simulink model "msync_foc"  (R2026a)
settings: Solver=ode15s  StopTime=t_sim  MaxStep=1e-4  MinStep=1e-8  RelTol=1e-4  AbsTol=1e-6
values from neighbouring files (symbols this model uses):
  f_frot = 1e-3    (= 0.001)    [init_machine_synchrone.m]
  Gamma_c = 1.0    (= 1)    [init_machine_synchrone.m]
  id_ref = 0    [init_machine_synchrone.m]
  Ir_ref = 4    [init_machine_synchrone.m]
  J = m*R^2/2    (= 0.246615023307)    [init_machine_synchrone.m]
  Ki_dq = Rs / tau_c    (= 1125)    [init_machine_synchrone.m]
  Ki_w = Kp_w / tau_w    (= 33891.230015)    [init_machine_synchrone.m]
  Kp_dq = Ls / tau_c    (= 15)    [init_machine_synchrone.m]
  Kp_w = J / (tau_w * M0 * Ir_ref)    (= 451.883066866)    [init_machine_synchrone.m]
  kr = ws_nom / t_rampe    (= 3.14159265359)    [init_machine_synchrone.m]
  Ls = 20e-3    (= 0.02)    [init_machine_synchrone.m]
  M0 = (V_ent/(2*mu0))*Ks*Kr    (= 0.010232805843)    [init_machine_synchrone.m]
  param_elec = [Rs ; Ls ; Rr ; Lr ; M0]    [init_machine_synchrone.m]
  Rr = 2.0    (= 2)    [init_machine_synchrone.m]
  theta0 = -pi/4    (= -0.785398163397)    [init_machine_synchrone.m]
  w0 = 0    [init_machine_synchrone.m]
  ws_nom = 2*pi*5    (= 31.4159265359)    [init_machine_synchrone.m]
  x_elec_0 = [i1_0; i2_0; Ir_0]    [init_machine_synchrone.m]
libraries: slpidlib x3, simulink x1
settings DebuggingCC: UnderSpecifiedDimensionMsg=warning

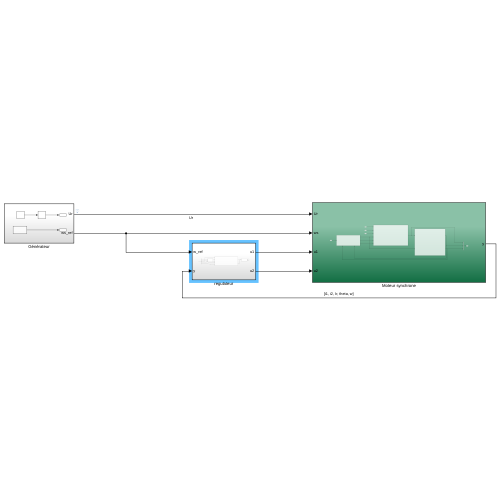
[thumbnail: Simulink's stored preview of the top-level diagram]
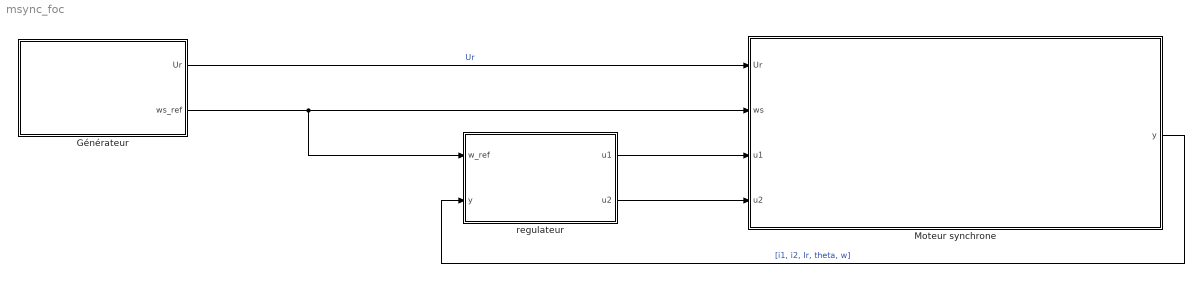
== system msync_foc ==
  Générateur : Subsystem
  Moteur synchrone : Subsystem
  regulateur : Subsystem
  wires:
  Générateur/1(Ur) -> Moteur synchrone/1(Ur)  "Ur"
  Générateur/2(ws_ref) -> Moteur synchrone/2(ws), regulateur/1(w_ref)
  regulateur/1(u1) -> Moteur synchrone/3(u1)
  regulateur/2(u2) -> Moteur synchrone/4(u2)
  Moteur synchrone/1(y) -> regulateur/2(y)  "[i1, i2, Ir, theta, w]"

== system msync_foc/Générateur ==
  Consigne rampe : simulink/Sources/Ramp  slope=kr  start=0  InitialOutput=20
  Constant : Constant  Value=Ir_ref/Rr
  Saturation : Saturate  UpperLimit=ws_nom  LowerLimit=-inf
  Ur : Outport
  ws_ref : Outport  Port=2
  wires:
  Constant/1 -> Ur/1
  Consigne rampe/1 -> Saturation/1
  Saturation/1 -> ws_ref/1

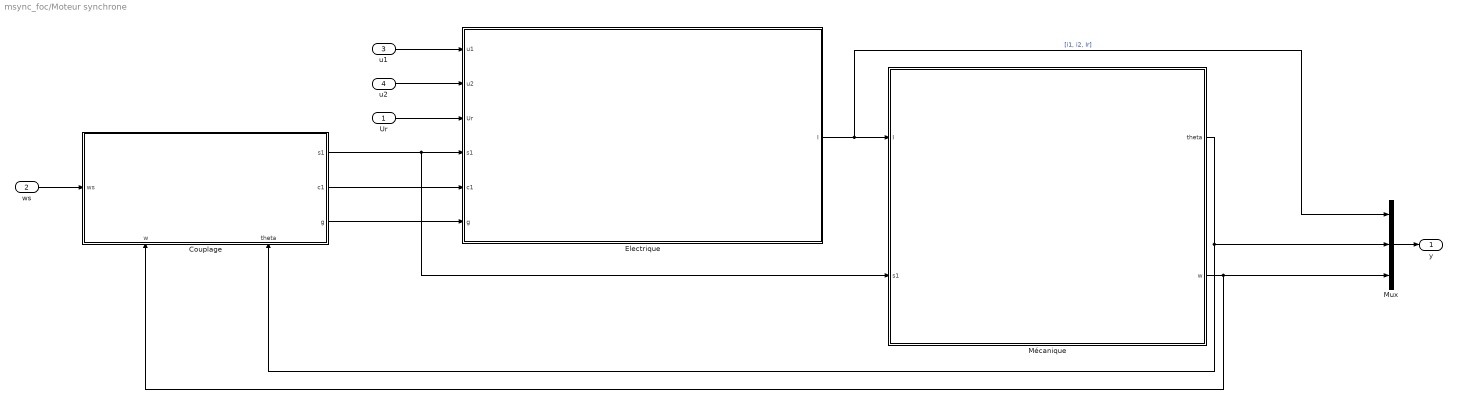
== system msync_foc/Moteur synchrone ==
  Ur : Inport
  ws : Inport  Port=2
  u1 : Inport  Port=3
  u2 : Inport  Port=4
  Couplage : Subsystem
      settings: PortSchema="{\"entries\":[{\"content\":{\"sides\":[{\"content\":{\"connectorIds\":[\"In1\"]},\"type\":\"ConnectorPlacement.EquallySpacedRectSide\",\"uuid\":\"9dc51e47-3ccd-4fcf-b58e-693782414d72\"},{\"content\":{\"connectorIds\":[\"Out1\",\"Out2\",\"Out3\"],\"side\":\"RIGHT\"},\"type\":\"ConnectorPlacement.EquallySpacedRectSide\",\"uuid\":\"19a88299-5411-4e53-b82f-2f137c46c168\"},{\"content\":{\"side\":\"TOP\"},\"type\":\"ConnectorPlacement.EquallySpacedRectSide\",\"uuid\":\"41370ab2-3a57-4936-8529-4b17c5065414\"},{\"content\":{\"connectorIds\":[\"In2\",\"In3\"],\"side\":\"BOTTOM\"},\"type\":\"ConnectorPlacement.EquallySpacedRectSide\",\"uuid\":\"3208a361-3d29-4bb8-a8eb-05b939f283cd\"}]},\"type\":\"ConnectorPlacement.EquallySpacedConnector\",\"uuid\":\"757f9aef-a381-4002-b608-7371e0c3c663\"}],\"packageUris\":[\"http://schema.mathworks.com/mf0/Connector/R2020b\"],\"version\":\"1.0\"}"
  Electrique : Subsystem
  Mux : Mux  Inputs=3
  Mécanique : Subsystem
  y : Outport
  wires:
  ws/1 -> Couplage/1(ws)
  Couplage/1(s1) -> Mécanique/2(s1), Electrique/4(s1)
  Couplage/3(g) -> Electrique/6(g)
  Mécanique/1(theta) -> Mux/2, Couplage/3(theta)
  Couplage/2(c1) -> Electrique/5(c1)
  Mécanique/2(w) -> Mux/3, Couplage/2(w)
  Ur/1 -> Electrique/3(Ur)
  u1/1 -> Electrique/1(u1)
  u2/1 -> Electrique/2(u2)
  Mux/1 -> y/1
  Electrique/1(I) -> Mux/1, Mécanique/1(I)  "[i1, i2, Ir]"

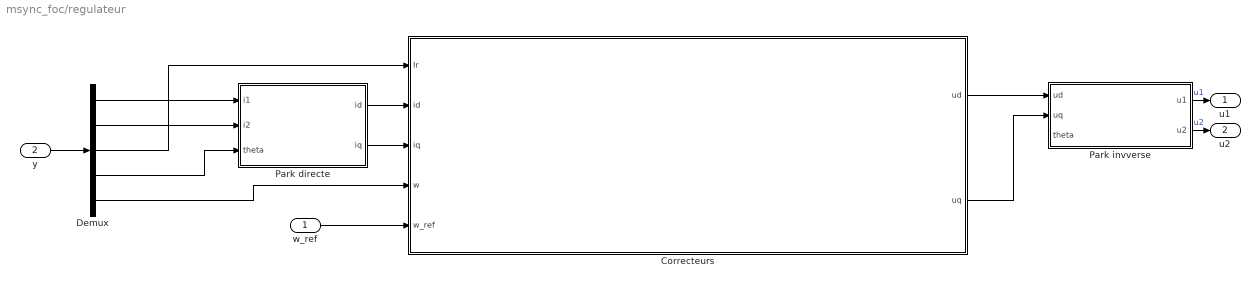
== system msync_foc/regulateur ==
  w_ref : Inport
  y : Inport  Port=2
  Correcteurs : Subsystem
  Demux : Demux  Outputs=5
  Park directe : Subsystem
  Park invverse : Subsystem
  u1 : Outport
  u2 : Outport  Port=2
  wires:
  w_ref/1 -> Correcteurs/5(w_ref)
  Park invverse/2(u2) -> u2/1  "u2"
  Park invverse/1(u1) -> u1/1  "u1"
  Demux/5 -> Correcteurs/4(w)
  Correcteurs/2(uq) -> Park invverse/2(uq)
  Correcteurs/1(ud) -> Park invverse/1(ud)
  Park directe/1(id) -> Correcteurs/2(id)
  Park directe/2(iq) -> Correcteurs/3(iq)
  y/1 -> Demux/1
  Demux/1 -> Park directe/1(i1)
  Demux/2 -> Park directe/2(i2)
  Demux/3 -> Correcteurs/1(Ir)
  Demux/4 -> Park directe/3(theta)

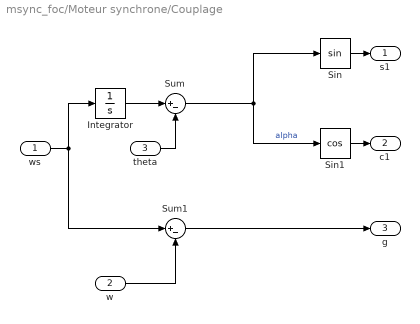
== system msync_foc/Moteur synchrone/Couplage ==
  ws : Inport
  w : Inport  Port=2
  theta : Inport  Port=3
  Integrator : Integrator
  Sin : Trigonometry
  Sin1 : Trigonometry  Operator=cos
  Sum : Sum  Inputs=|+-
  Sum1 : Sum  Inputs=|+-
  s1 : Outport
  c1 : Outport  Port=2
  g : Outport  Port=3
  wires:
  ws/1 -> Sum1/1, Integrator/1
  theta/1 -> Sum/2
  Integrator/1 -> Sum/1
  w/1 -> Sum1/2
  Sum/1 -> Sin1/1, Sin/1  "alpha"
  Sum1/1 -> g/1
  Sin/1 -> s1/1
  Sin1/1 -> c1/1

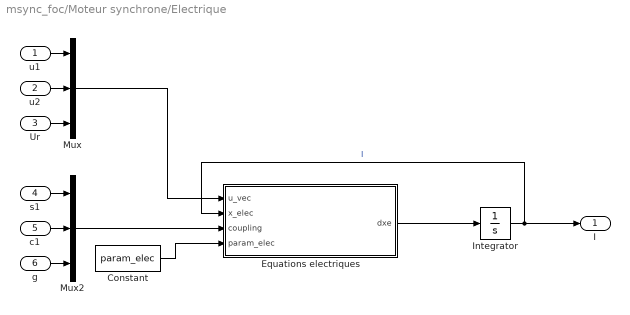
== system msync_foc/Moteur synchrone/Electrique ==
  u1 : Inport
  u2 : Inport  Port=2
  Ur : Inport  Port=3
  s1 : Inport  Port=4
  c1 : Inport  Port=5
  g : Inport  Port=6
  Constant : Constant  Value=param_elec
  Equations electriques : MATLAB Function  TreatAsAtomicUnit=on
  Integrator : Integrator  InitialCondition=x_elec_0'
  Mux : Mux  Inputs=3
  Mux2 : Mux  Inputs=3
  I : Outport
  wires:
  s1/1 -> Mux2/1
  Equations electriques/1(dxe) -> Integrator/1
  Mux2/1 -> Equations electriques/3(coupling)
  c1/1 -> Mux2/2
  Mux/1 -> Equations electriques/1(u_vec)
  u1/1 -> Mux/1
  u2/1 -> Mux/2
  Ur/1 -> Mux/3
  g/1 -> Mux2/3
  Constant/1 -> Equations electriques/4(param_elec)
  Integrator/1 -> I/1, Equations electriques/2(x_elec)  "I"

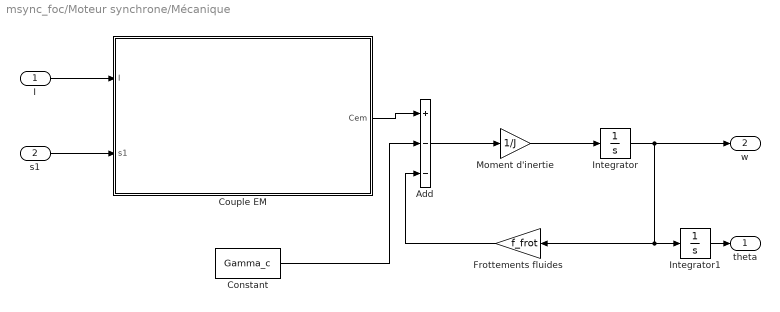
== system msync_foc/Moteur synchrone/Mécanique ==
  I : Inport
  s1 : Inport  Port=2
  Add : Sum  Inputs=+--
  Constant : Constant  Value=Gamma_c
  Couple EM : Subsystem
  Frottements fluides : Gain  Gain=f_frot
  Integrator : Integrator  InitialCondition=w0
  Integrator1 : Integrator  InitialCondition=theta0
  Moment d'inertie : Gain  Gain=1/J
  theta : Outport
  w : Outport  Port=2
  wires:
  Integrator/1 -> w/1, Integrator1/1, Frottements fluides/1
  I/1 -> Couple EM/1(I)
  Add/1 -> Moment d'inertie/1
  Moment d'inertie/1 -> Integrator/1
  Frottements fluides/1 -> Add/3
  s1/1 -> Couple EM/2(s1)
  Integrator1/1 -> theta/1
  Constant/1 -> Add/2
  Couple EM/1(Cem) -> Add/1

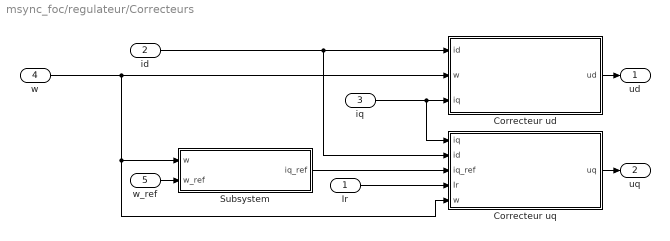
== system msync_foc/regulateur/Correcteurs ==
  Ir : Inport
  id : Inport  Port=2
  iq : Inport  Port=3
  w : Inport  Port=4
  w_ref : Inport  Port=5
  Correcteur ud : Subsystem
  Correcteur uq : Subsystem
  Subsystem : Subsystem
  ud : Outport
  uq : Outport  Port=2
  wires:
  Ir/1 -> Correcteur uq/4(Ir)
  id/1 -> Correcteur ud/1(id), Correcteur uq/2(id)
  w/1 -> Correcteur uq/5(w), Subsystem/1(w), Correcteur ud/2(w)
  Correcteur ud/1(ud) -> ud/1
  iq/1 -> Correcteur uq/1(iq), Correcteur ud/3(iq)
  Subsystem/1(iq_ref) -> Correcteur uq/3(iq_ref)
  Correcteur uq/1(uq) -> uq/1
  w_ref/1 -> Subsystem/2(w_ref)

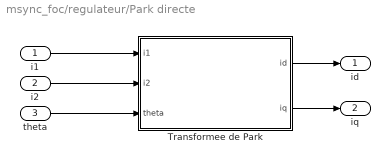
== system msync_foc/regulateur/Park directe ==
  i1 : Inport
  i2 : Inport  Port=2
  theta : Inport  Port=3
  Transformee de Park : MATLAB Function  TreatAsAtomicUnit=on
  id : Outport
  iq : Outport  Port=2
  wires:
  i1/1 -> Transformee de Park/1(i1)
  theta/1 -> Transformee de Park/3(theta)
  i2/1 -> Transformee de Park/2(i2)
  Transformee de Park/1(id) -> id/1
  Transformee de Park/2(iq) -> iq/1

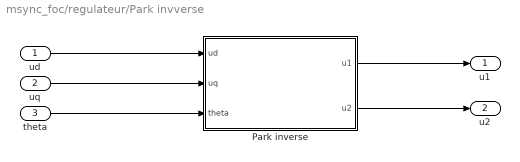
== system msync_foc/regulateur/Park invverse ==
  ud : Inport
  uq : Inport  Port=2
  theta : Inport  Port=3
  Park inverse : MATLAB Function  TreatAsAtomicUnit=on
  u1 : Outport
  u2 : Outport  Port=2
  wires:
  theta/1 -> Park inverse/3(theta)
  uq/1 -> Park inverse/2(uq)
  ud/1 -> Park inverse/1(ud)
  Park inverse/1(u1) -> u1/1
  Park inverse/2(u2) -> u2/1

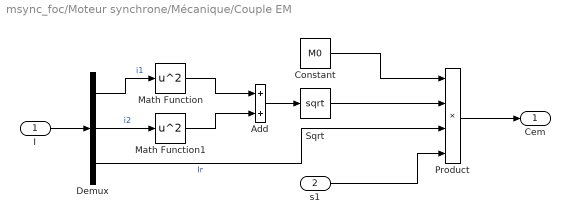
== system msync_foc/Moteur synchrone/Mécanique/Couple EM ==
  I : Inport
  s1 : Inport  Port=2
  Add : Sum
  Constant : Constant  Value=M0
  Demux : Demux  Outputs=3
  Math Function : Math  Operator=square
  Math Function1 : Math  Operator=square
  Product : Product  Inputs=4
  Sqrt : Sqrt
  Cem : Outport
  wires:
  Math Function/1 -> Add/1
  Math Function1/1 -> Add/2
  Add/1 -> Sqrt/1
  I/1 -> Demux/1
  Product/1 -> Cem/1
  Sqrt/1 -> Product/2
  Constant/1 -> Product/1
  s1/1 -> Product/4
  Demux/3 -> Product/3  "Ir"
  Demux/2 -> Math Function1/1  "i2"
  Demux/1 -> Math Function/1  "i1"

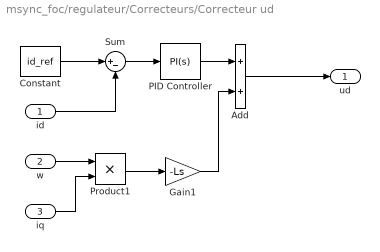
== system msync_foc/regulateur/Correcteurs/Correcteur ud ==
  id : Inport
  w : Inport  Port=2
  iq : Inport  Port=3
  Add : Sum
  Constant : Constant  Value=id_ref
  Gain1 : Gain  Gain=-Ls
  PID Controller : slpidlib/PID Controller  Controller=PI  Form=Parallel  TimeDomain=Continuous-time  UseExternalTs=off  SampleTime=-1  IntegratorMethod=Forward Euler  FilterMethod=Forward Euler  ControllerParametersSource=internal  P=Kp_dq  I=Ki_dq  UseKiTs=off  D=0  UseExternalDerivativeSource=off  N=100  UseFilter=on  TunerSelectOption=Transfer Function Based (PID Tuner App)  InitialConditionSource=internal  InitialConditionForIntegrator=0  InitialConditionForFilter=0  DifferentiatorICPrevScaledInput=0  ExternalReset=none  TrackingMode=off  Kt=1  LimitOutput=off  SatLimitsSource=internal  UpperSaturationLimit=inf  LowerSaturationLimit=-inf  LinearizeAsGain=on  AntiWindupMode=none  Kb=1  LimitIntegrator=off  UpperIntegratorSaturationLimit=inf  LowerIntegratorSaturationLimit=-inf  POutMin=[]  POutMax=[]  IOutMin=[]  IOutMax=[]  DOutMin=[]  DOutMax=[]  NOutMin=[]  NOutMax=[]  SumOutMin=[]  SumOutMax=[]  SaturationOutMin=[]  SaturationOutMax=[]  PParamMin=[]  PParamMax=[]  IParamMin=[]  IParamMax=[]  DParamMin=[]  DParamMax=[]  NParamMin=[]  NParamMax=[]  KbParamMin=[]  KbParamMax=[]  KtParamMin=[]  KtParamMax=[]  KbOutMin=[]  KbOutMax=[]  KtOutMin=[]  KtOutMax=[]  IntegratorOutMin=[]  IntegratorOutMax=[]  FilterOutMin=[]  FilterOutMax=[]  SumI1OutMin=[]  SumI1OutMax=[]  SumI2OutMin=[]  SumI2OutMax=[]  SumI3OutMin=[]  SumI3OutMax=[]  SumI4OutMin=[]  SumI4OutMax=[]  SumDOutMin=[]  SumDOutMax=[]  DifferentiatorOutMin=[]  DifferentiatorOutMax=[]  FilterDiffOutCoefMin=[]  FilterDiffOutCoefMax=[]  ReciprocalOutMin=[]  ReciprocalOutMax=[]  SumDenOutMin=[]  SumDenOutMax=[]  SumNumOutMin=[]  SumNumOutMax=[]  DivideOutMin=[]  DivideOutMax=[]  UdiffTsProdOutMin=[]  UdiffTsProdOutMax=[]  NTsProdOutMin=[]  NTsProdOutMax=[]  UintegralTsProdOutMin=[]  UintegralTsProdOutMax=[]  UngainTsProdOutMin=[]  UngainTsProdOutMax=[]  ClampingZeroOutDataTypeStr=Inherit: Inherit via back propagation  ClampingZeroOutMin=[]  ClampingZeroOutMax=[]  FilterDenConstantOutDataTypeStr=Inherit: Inherit via back propagation  FilterDenConstantOutMin=[]  FilterDenConstantOutMax=[]  PCopyOutDataTypeStr=Inherit: Inherit via back propagation  PCopyOutMin=[]  PCopyOutMax=[]  NCopyOutDataTypeStr=Inherit: Inherit via back propagation  NCopyOutMin=[]  NCopyOutMax=[]  IntegratorContinuousStateAttributes=''  IntegratorStateMustResolveToSignalObject=off  IntegratorRTWStateStorageClass=Auto  FilterContinuousStateAttributes=''  FilterStateMustResolveToSignalObject=off  FilterRTWStateStorageClass=Auto  ParallelPVariant=InternalParameters  IdealPVariant=Disabled  IVariant=InternalParameters  DVariant=Disabled  IntegratorVariant=Continuous  SatVariant=Disabled  AWVariant=Passthrough  PCopyVariant=Disabled  TRVariant=Disabled  FdbkBlocksVariant=Forward  IdealPFdbkVariant=Disabled  SatFdbkVariant=Disabled  DerivativeFilterVariant=Disabled  NVariant=Disabled  NCopyVariant=Disabled_SignalSpec  FilterICVariant=Disabled  IntegratorICVariant=InternalICs  ExternalResetVariant=Disabled  TRSumVariant=Passthrough  SumFdbkVariant=Disabled  SumVariant=Sum_PI  TsampFilterVariant=InternalTs  TsampNgainVariant=Passthrough  TsampIntegralVariant=Disabled_SignalSpec  ExternalSaturationOutDataTypeStr=Inherit: Same as second input  DerivativeSourceVariant=Disabled  PreIntVariant=InternalPreInt
  Product1 : Product
  Sum : Sum  Inputs=|+-
  ud : Outport
  wires:
  Constant/1 -> Sum/1
  Sum/1 -> PID Controller/1
  id/1 -> Sum/2
  PID Controller/1 -> Add/1
  Add/1 -> ud/1
  iq/1 -> Product1/2
  w/1 -> Product1/1
  Product1/1 -> Gain1/1
  Gain1/1 -> Add/2

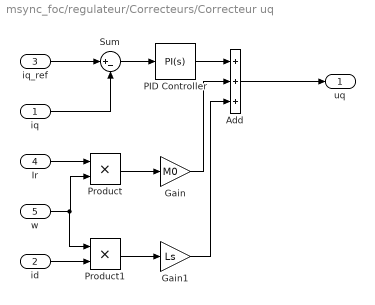
== system msync_foc/regulateur/Correcteurs/Correcteur uq ==
  iq : Inport
  id : Inport  Port=2
  iq_ref : Inport  Port=3
  Ir : Inport  Port=4
  w : Inport  Port=5
  Add : Sum  Inputs=+++
  Gain : Gain  Gain=M0
  Gain1 : Gain  Gain=Ls
  PID Controller : slpidlib/PID Controller  Controller=PI  Form=Parallel  TimeDomain=Continuous-time  UseExternalTs=off  SampleTime=-1  IntegratorMethod=Forward Euler  FilterMethod=Forward Euler  ControllerParametersSource=internal  P=Kp_dq  I=Ki_dq  UseKiTs=off  D=0  UseExternalDerivativeSource=off  N=100  UseFilter=on  TunerSelectOption=Transfer Function Based (PID Tuner App)  InitialConditionSource=internal  InitialConditionForIntegrator=0  InitialConditionForFilter=0  DifferentiatorICPrevScaledInput=0  ExternalReset=none  TrackingMode=off  Kt=1  LimitOutput=off  SatLimitsSource=internal  UpperSaturationLimit=inf  LowerSaturationLimit=-inf  LinearizeAsGain=on  AntiWindupMode=none  Kb=1  LimitIntegrator=off  UpperIntegratorSaturationLimit=inf  LowerIntegratorSaturationLimit=-inf  POutMin=[]  POutMax=[]  IOutMin=[]  IOutMax=[]  DOutMin=[]  DOutMax=[]  NOutMin=[]  NOutMax=[]  SumOutMin=[]  SumOutMax=[]  SaturationOutMin=[]  SaturationOutMax=[]  PParamMin=[]  PParamMax=[]  IParamMin=[]  IParamMax=[]  DParamMin=[]  DParamMax=[]  NParamMin=[]  NParamMax=[]  KbParamMin=[]  KbParamMax=[]  KtParamMin=[]  KtParamMax=[]  KbOutMin=[]  KbOutMax=[]  KtOutMin=[]  KtOutMax=[]  IntegratorOutMin=[]  IntegratorOutMax=[]  FilterOutMin=[]  FilterOutMax=[]  SumI1OutMin=[]  SumI1OutMax=[]  SumI2OutMin=[]  SumI2OutMax=[]  SumI3OutMin=[]  SumI3OutMax=[]  SumI4OutMin=[]  SumI4OutMax=[]  SumDOutMin=[]  SumDOutMax=[]  DifferentiatorOutMin=[]  DifferentiatorOutMax=[]  FilterDiffOutCoefMin=[]  FilterDiffOutCoefMax=[]  ReciprocalOutMin=[]  ReciprocalOutMax=[]  SumDenOutMin=[]  SumDenOutMax=[]  SumNumOutMin=[]  SumNumOutMax=[]  DivideOutMin=[]  DivideOutMax=[]  UdiffTsProdOutMin=[]  UdiffTsProdOutMax=[]  NTsProdOutMin=[]  NTsProdOutMax=[]  UintegralTsProdOutMin=[]  UintegralTsProdOutMax=[]  UngainTsProdOutMin=[]  UngainTsProdOutMax=[]  ClampingZeroOutDataTypeStr=Inherit: Inherit via back propagation  ClampingZeroOutMin=[]  ClampingZeroOutMax=[]  FilterDenConstantOutDataTypeStr=Inherit: Inherit via back propagation  FilterDenConstantOutMin=[]  FilterDenConstantOutMax=[]  PCopyOutDataTypeStr=Inherit: Inherit via back propagation  PCopyOutMin=[]  PCopyOutMax=[]  NCopyOutDataTypeStr=Inherit: Inherit via back propagation  NCopyOutMin=[]  NCopyOutMax=[]  IntegratorContinuousStateAttributes=''  IntegratorStateMustResolveToSignalObject=off  IntegratorRTWStateStorageClass=Auto  FilterContinuousStateAttributes=''  FilterStateMustResolveToSignalObject=off  FilterRTWStateStorageClass=Auto  ParallelPVariant=InternalParameters  IdealPVariant=Disabled  IVariant=InternalParameters  DVariant=Disabled  IntegratorVariant=Continuous  SatVariant=Disabled  AWVariant=Passthrough  PCopyVariant=Disabled  TRVariant=Disabled  FdbkBlocksVariant=Forward  IdealPFdbkVariant=Disabled  SatFdbkVariant=Disabled  DerivativeFilterVariant=Disabled  NVariant=Disabled  NCopyVariant=Disabled_SignalSpec  FilterICVariant=Disabled  IntegratorICVariant=InternalICs  ExternalResetVariant=Disabled  TRSumVariant=Passthrough  SumFdbkVariant=Disabled  SumVariant=Sum_PI  TsampFilterVariant=InternalTs  TsampNgainVariant=Passthrough  TsampIntegralVariant=Disabled_SignalSpec  ExternalSaturationOutDataTypeStr=Inherit: Same as second input  DerivativeSourceVariant=Disabled  PreIntVariant=InternalPreInt
  Product : Product
  Product1 : Product
  Sum : Sum  Inputs=|+-
  uq : Outport
  wires:
  iq_ref/1 -> Sum/1
  Sum/1 -> PID Controller/1
  iq/1 -> Sum/2
  PID Controller/1 -> Add/1
  Add/1 -> uq/1
  Product/1 -> Gain/1
  Ir/1 -> Product/1
  id/1 -> Product1/2
  w/1 -> Product1/1, Product/2
  Product1/1 -> Gain1/1
  Gain1/1 -> Add/3
  Gain/1 -> Add/2

== system msync_foc/regulateur/Correcteurs/Subsystem ==
  w : Inport
  w_ref : Inport  Port=2
  PID Controller : slpidlib/PID Controller  Controller=PI  Form=Parallel  TimeDomain=Continuous-time  UseExternalTs=off  SampleTime=-1  IntegratorMethod=Forward Euler  FilterMethod=Forward Euler  ControllerParametersSource=internal  P=Kp_w  I=Ki_w  UseKiTs=off  D=0  UseExternalDerivativeSource=off  N=100  UseFilter=on  TunerSelectOption=Transfer Function Based (PID Tuner App)  InitialConditionSource=internal  InitialConditionForIntegrator=0  InitialConditionForFilter=0  DifferentiatorICPrevScaledInput=0  ExternalReset=none  TrackingMode=off  Kt=1  LimitOutput=off  SatLimitsSource=internal  UpperSaturationLimit=inf  LowerSaturationLimit=-inf  LinearizeAsGain=on  AntiWindupMode=none  Kb=1  LimitIntegrator=off  UpperIntegratorSaturationLimit=inf  LowerIntegratorSaturationLimit=-inf  POutMin=[]  POutMax=[]  IOutMin=[]  IOutMax=[]  DOutMin=[]  DOutMax=[]  NOutMin=[]  NOutMax=[]  SumOutMin=[]  SumOutMax=[]  SaturationOutMin=[]  SaturationOutMax=[]  PParamMin=[]  PParamMax=[]  IParamMin=[]  IParamMax=[]  DParamMin=[]  DParamMax=[]  NParamMin=[]  NParamMax=[]  KbParamMin=[]  KbParamMax=[]  KtParamMin=[]  KtParamMax=[]  KbOutMin=[]  KbOutMax=[]  KtOutMin=[]  KtOutMax=[]  IntegratorOutMin=[]  IntegratorOutMax=[]  FilterOutMin=[]  FilterOutMax=[]  SumI1OutMin=[]  SumI1OutMax=[]  SumI2OutMin=[]  SumI2OutMax=[]  SumI3OutMin=[]  SumI3OutMax=[]  SumI4OutMin=[]  SumI4OutMax=[]  SumDOutMin=[]  SumDOutMax=[]  DifferentiatorOutMin=[]  DifferentiatorOutMax=[]  FilterDiffOutCoefMin=[]  FilterDiffOutCoefMax=[]  ReciprocalOutMin=[]  ReciprocalOutMax=[]  SumDenOutMin=[]  SumDenOutMax=[]  SumNumOutMin=[]  SumNumOutMax=[]  DivideOutMin=[]  DivideOutMax=[]  UdiffTsProdOutMin=[]  UdiffTsProdOutMax=[]  NTsProdOutMin=[]  NTsProdOutMax=[]  UintegralTsProdOutMin=[]  UintegralTsProdOutMax=[]  UngainTsProdOutMin=[]  UngainTsProdOutMax=[]  ClampingZeroOutDataTypeStr=Inherit: Inherit via back propagation  ClampingZeroOutMin=[]  ClampingZeroOutMax=[]  FilterDenConstantOutDataTypeStr=Inherit: Inherit via back propagation  FilterDenConstantOutMin=[]  FilterDenConstantOutMax=[]  PCopyOutDataTypeStr=Inherit: Inherit via back propagation  PCopyOutMin=[]  PCopyOutMax=[]  NCopyOutDataTypeStr=Inherit: Inherit via back propagation  NCopyOutMin=[]  NCopyOutMax=[]  IntegratorContinuousStateAttributes=''  IntegratorStateMustResolveToSignalObject=off  IntegratorRTWStateStorageClass=Auto  FilterContinuousStateAttributes=''  FilterStateMustResolveToSignalObject=off  FilterRTWStateStorageClass=Auto  ParallelPVariant=InternalParameters  IdealPVariant=Disabled  IVariant=InternalParameters  DVariant=Disabled  IntegratorVariant=Continuous  SatVariant=Disabled  AWVariant=Passthrough  PCopyVariant=Disabled  TRVariant=Disabled  FdbkBlocksVariant=Forward  IdealPFdbkVariant=Disabled  SatFdbkVariant=Disabled  DerivativeFilterVariant=Disabled  NVariant=Disabled  NCopyVariant=Disabled_SignalSpec  FilterICVariant=Disabled  IntegratorICVariant=InternalICs  ExternalResetVariant=Disabled  TRSumVariant=Passthrough  SumFdbkVariant=Disabled  SumVariant=Sum_PI  TsampFilterVariant=InternalTs  TsampNgainVariant=Passthrough  TsampIntegralVariant=Disabled_SignalSpec  ExternalSaturationOutDataTypeStr=Inherit: Same as second input  DerivativeSourceVariant=Disabled  PreIntVariant=InternalPreInt
  Sum : Sum  Inputs=|+-
  iq_ref : Outport
  wires:
  w_ref/1 -> Sum/1
  Sum/1 -> PID Controller/1
  w/1 -> Sum/2
  PID Controller/1 -> iq_ref/1

== matlab function msync_foc/regulateur/Park directe/Transformee de Park ==
  data: i1 input size=1; i2 input size=1; id output size=1; theta input size=1; iq output size=1
function [id, iq] = park_transform(i1, i2, theta)

cost = cos(theta);
sint = sin(theta);

id = cost * i1 + sint * i2;
iq = -sint * i1 + cost * i2;

== matlab function msync_foc/Moteur synchrone/Electrique/Equations electriques ==
  data: u_vec input size=[1 3]; dxe output size=[1 3]; x_elec input size=[1 3]; coupling input size=[1 3]; param_elec input size=[1 5]
function dxe = electrical_equations(u_vec, x_elec, coupling, param_elec)

% Importation des parametres depuis la workspace
Rs = param_elec(1);
Ls = param_elec(2);
Rr = param_elec(3);
Lr = param_elec(4);
M0 = param_elec(5);

% Extraction des signaux
u1 = u_vec(1); u2 = u_vec(2); Ur = u_vec(3);
i1 = x_elec(1); i2 = x_elec(2); Ir = x_elec(3);
s1 = coupling(1); % sin(ws*t-theta)
c1 = coupling(2); % cos(ws*t-theta)
g  = coupling(3); % ws*t - omega

Ism = sqrt(i1^2+i2^2);

% Phase statorique 1
di1 = (u1-Rs*i1-M0*Ir*g*s1)/Ls;

% Phase statorique 2
% Note: +cos car sin(ws*t-theta+pi/2) = cos(ws*t-theta)
di2 = (u2-Rs*i2+M0*Ir*g*c1)/Ls;

% Circuit rotorique
dIr = (Ur-Rr*Ir-M0*Ism*g*(-s1))/Lr;

dxe = [di1, di2, dIr];

== matlab function msync_foc/regulateur/Park invverse/Park inverse ==
  data: ud input size=1; uq input size=1; u1 output size=1; theta input size=1; u2 output size=1
function [u1, u2] = park_inverse(ud, uq, theta)

cost = cos(theta);
sint = sin(theta);

u1 = cost * ud - sint * uq;
u2 = sint * ud + cost * uq;
